simulink model "flexibleBody_lib_example"  (R2018b)
settings: Solver=VariableStepAuto  StartTime=0.0  StopTime=10.0  RelTol=1e-3
values from neighbouring files (symbols this model uses):
  structure = structureCreate( 'structure_params_default' )    [flexibleBody_lib_example_init.m]
  structure_red = structureGetReduced(structure,num_modes)    [flexibleBody_lib_example_init.m]
undefined symbols (not defined in the file or in its folder): structureGetNodeCg, structureGetNodeMass, structureGetTotalInertia, structureGetTotalMass
libraries: flexibleBody_lib x1
settings Model: Creator=yannic  LastModifiedBy=yannic

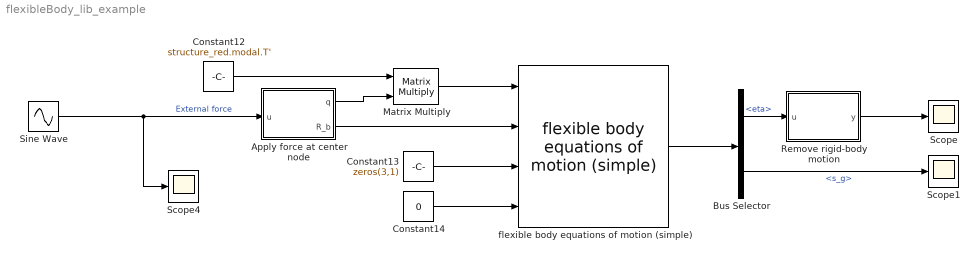
== system flexibleBody_lib_example ==
  Apply force at center node : MATLAB Function  TreatAsAtomicUnit=on
  Bus Selector : BusSelector  OutputSignals=eta,rigidBodyBus.s_g
  Constant12 : Constant  Value=structure_red.modal.T'
  Constant13 : Constant  Value=zeros(3,1)
  Constant14 : Constant  Value=0
  Matrix Multiply : Product  Multiplication=Matrix(*)
  Remove rigid-body motion : MATLAB Function  TreatAsAtomicUnit=on
  Scope : Scope
  Scope1 : Scope
  Scope4 : Scope
  Sine Wave : Sin  SampleTime=0
  flexible body equations of motion (simple) : flexibleBody_lib/flexible body equations of motion (simple)  structure_red=structure_red  m=structureGetTotalMass(structure)  I_b=structureGetTotalInertia(structure)  m_nodes=structureGetNodeMass(structure,1:length(structure.xyz))  cg_nodes=structureGetNodeCg(structure,1:length(structure.xyz))  structure_vel_0=zeros(size(structure_red.K,2)-6,1)  structure_pos_0=zeros(size(structure_red.K,2)-6,1)
      settings: SourceProductName=LADAC
  wires:
  Constant14/1 -> flexible body equations of motion (simple)/4
  Constant12/1 -> Matrix Multiply/1
  Apply force at center node/1(q) -> Matrix Multiply/2
  Apply force at center node/2(R_b) -> flexible body equations of motion (simple)/2
  Matrix Multiply/1 -> flexible body equations of motion (simple)/1
  Sine Wave/1 -> Scope4/1, Apply force at center node/1(u)  "External force"
  Constant13/1 -> flexible body equations of motion (simple)/3
  flexible body equations of motion (simple)/1 -> Bus Selector/1
  Bus Selector/1 -> Remove rigid-body motion/1(u)  "<eta>"
  Bus Selector/2 -> Scope1/1  "<s_g>"
  Remove rigid-body motion/1(y) -> Scope/1

== matlab function flexibleBody_lib_example/Remove rigid-body motion ==
  data: u input; y output
function y = fcn(u)
y = u(7:end);
end

== matlab function flexibleBody_lib_example/Apply force at center node ==
  data: u input; q output; R_b output; structure parameter
function [q,R_b] = fcn(u,structure)
num_nodes = size(structure.xyz,2);
q = zeros(6*num_nodes,1);
q((num_nodes/2-0.5)*6+3) = u;
R_b = zeros(3,1);
R_b(3) = u;
end
